simulink model "sim_MRAC_Plant"  (Simulink 7.2)
settings: Solver=ode3  StartTime=0.0  StopTime=10.0  FixedStep=ts  RelTol=1e-3
undefined symbols (not defined in the file or in its folder): ka, kq, Ma, Md, Mq, Za, Zd
settings Model: Creator=E183308  LastModifiedBy=E183308
settings OptimizationCC: InitFltsAndDblsToZero=on
settings DebuggingCC: SaveWithParameterizedLinksMsg=none  SignalResolutionControl=TryResolveAllWithWarning  MultiTaskDSMMsg=warning  MultiTaskCondExecSysMsg=none
settings RTWCC: IncludeERTFirstTime=on
settings GRTTargetCC: TargetFcnLib=ansi_tfl_tmw.mat

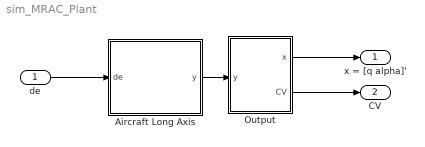
== system sim_MRAC_Plant ==
  de : Inport  OutDataType=sfix(16)  OutScaling=2^0
  Aircraft Long Axis : Subsystem
  Output : Subsystem
  x = [q alpha]' : Outport  OutDataType=sfix(16)  OutScaling=2^0
  CV : Outport  Port=2  OutDataType=sfix(16)  OutScaling=2^0
  wires:
  Output/2(CV) -> CV/1
  Output/1(x) -> x = [q alpha]'/1
  de/1 -> Aircraft Long Axis/1(de)
  Aircraft Long Axis/1(y) -> Output/1(y)

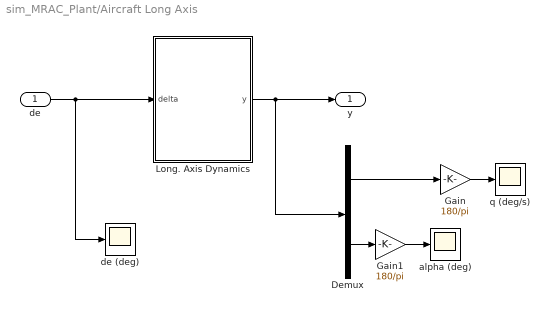
== system sim_MRAC_Plant/Aircraft Long Axis ==
  de : Inport  OutDataType=sfix(16)  OutScaling=2^0
  Demux : Demux  Outputs=[1 1]
  Gain : Gain  Gain=180/pi  ParameterDataType=sfix(16)  ParameterScaling=2^0  OutDataType=sfix(16)  OutScaling=2^0
  Gain1 : Gain  Gain=180/pi  ParameterDataType=sfix(16)  ParameterScaling=2^0  OutDataType=sfix(16)  OutScaling=2^0
  Long. Axis Dynamics : Subsystem
  alpha (deg) : Scope
      settings: TimeRange=10  YMin=0  SaveName=ScopeData10
  de (deg) : Scope
      settings: TimeRange=10  YMin=-20  YMax=20  SaveName=ScopeData3
  q (deg/s) : Scope
      settings: TimeRange=10  YMin=0  SaveName=ScopeData2
  y : Outport  OutDataType=sfix(16)  OutScaling=2^0
  wires:
  Long. Axis Dynamics/1(y) -> y/1, Demux/1
  Gain/1 -> q (deg/s)/1
  de/1 -> Long. Axis Dynamics/1(delta), de (deg)/1
  Gain1/1 -> alpha (deg)/1
  Demux/2 -> Gain1/1
  Demux/1 -> Gain/1

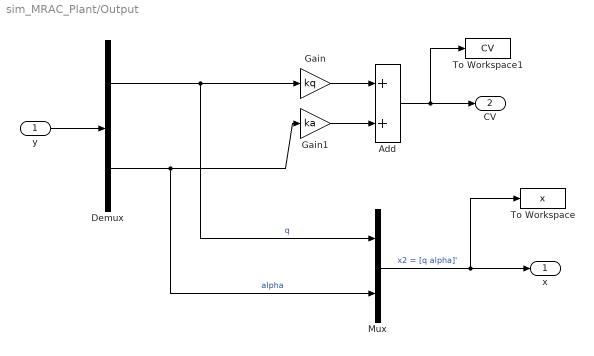
== system sim_MRAC_Plant/Output ==
  y : Inport  OutDataType=sfix(16)  OutScaling=2^0
  Add : Sum  OutDataType=sfix(16)  OutScaling=2^-10
  Demux : Demux  Outputs=[1 1]
  Gain : Gain  Gain=kq  ParameterDataType=sfix(16)  ParameterScaling=2^0  OutDataType=sfix(16)  OutScaling=2^0
  Gain1 : Gain  Gain=ka  ParameterDataType=sfix(16)  ParameterScaling=2^0  OutDataType=sfix(16)  OutScaling=2^0
  Mux : Mux  Inputs=[1 1]
  To Workspace : ToWorkspace  VariableName=x  SampleTime=-1  SaveFormat=Array
  To Workspace1 : ToWorkspace  VariableName=CV  SampleTime=-1  SaveFormat=Array
  x : Outport  OutDataType=sfix(16)  OutScaling=2^0
  CV : Outport  Port=2  OutDataType=sfix(16)  OutScaling=2^0
  wires:
  Mux/1 -> x/1, To Workspace/1  "x2 = [q alpha]'"
  y/1 -> Demux/1
  Gain/1 -> Add/1
  Gain1/1 -> Add/2
  Add/1 -> CV/1, To Workspace1/1
  Demux/1 -> Gain/1, Mux/1  "q"
  Demux/2 -> Gain1/1, Mux/2  "alpha"

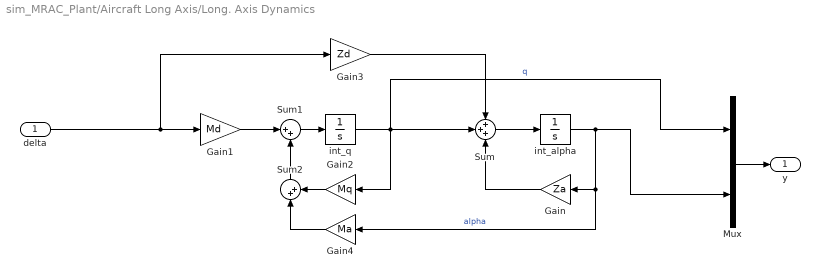
== system sim_MRAC_Plant/Aircraft Long Axis/Long. Axis Dynamics ==
  delta : Inport  OutDataType=sfix(16)  OutScaling=2^0
  Gain : Gain  Orientation=left  Gain=Za  ParameterDataType=sfix(16)  ParameterScaling=2^0  OutDataType=sfix(16)  OutScaling=2^0  SaturateOnIntegerOverflow=on  OutDataTypeStr=Inherit: Same as input  ParamDataTypeStr=Inherit: Same as input
  Gain1 : Gain  Gain=Md  ParameterDataType=sfix(16)  ParameterScaling=2^0  OutDataType=sfix(16)  OutScaling=2^0  SaturateOnIntegerOverflow=on  OutDataTypeStr=Inherit: Same as input  ParamDataTypeStr=Inherit: Same as input
  Gain2 : Gain  Orientation=left  Gain=Mq  ParameterDataType=sfix(16)  ParameterScaling=2^0  OutDataType=sfix(16)  OutScaling=2^0  SaturateOnIntegerOverflow=on  OutDataTypeStr=Inherit: Same as input  ParamDataTypeStr=Inherit: Same as input
  Gain3 : Gain  Gain=Zd  ParameterDataType=sfix(16)  ParameterScaling=2^0  OutDataType=sfix(16)  OutScaling=2^0  SaturateOnIntegerOverflow=on  OutDataTypeStr=Inherit: Same as input  ParamDataTypeStr=Inherit: Same as input
  Gain4 : Gain  Orientation=left  Gain=Ma  ParameterDataType=sfix(16)  ParameterScaling=2^0  OutDataType=sfix(16)  OutScaling=2^0  SaturateOnIntegerOverflow=on  OutDataTypeStr=Inherit: Same as input  ParamDataTypeStr=Inherit: Same as input
  Mux : Mux  Inputs=2
  Sum : Sum  Inputs=+++  OutDataType=sfix(16)  OutScaling=2^0  SaturateOnIntegerOverflow=on  InputSameDT=on  OutDataTypeStr=Inherit: Same as first input
  Sum1 : Sum  Inputs=|++  OutDataType=sfix(16)  OutScaling=2^0  SaturateOnIntegerOverflow=on  InputSameDT=on  OutDataTypeStr=Inherit: Same as first input
  Sum2 : Sum  Orientation=up  Inputs=|++  OutDataType=sfix(16)  OutScaling=2^0  SaturateOnIntegerOverflow=on  InputSameDT=on  OutDataTypeStr=Inherit: Same as first input
  int_alpha : Integrator
  int_q : Integrator
  y : Outport  OutDataType=sfix(16)  OutScaling=2^0
  wires:
  Mux/1 -> y/1
  Gain4/1 -> Sum2/1
  Sum2/1 -> Sum1/2
  Gain2/1 -> Sum2/2
  Gain3/1 -> Sum/1
  Gain1/1 -> Sum1/1
  Sum1/1 -> int_q/1
  int_alpha/1 -> Gain/1, Gain4/1, Mux/2  "alpha"
  Sum/1 -> int_alpha/1
  Gain/1 -> Sum/3
  int_q/1 -> Gain2/1, Mux/1, Sum/2  "q"
  delta/1 -> Gain1/1, Gain3/1
